simulink model "protocol"  (R2021b)
settings: Solver=FixedStepAuto  StartTime=0.0  StopTime=10.0  RelTol=1e-3
settings Model: Creator=marco  LastModifiedBy=makev
settings ModelReferenceCC: UpdateModelReferenceTargets=IfOutOfDate
settings ConfigComp: DVTestSuiteOptimization=Auto  DVDetectOutOfBounds=on  DVModelReferenceHarness=on

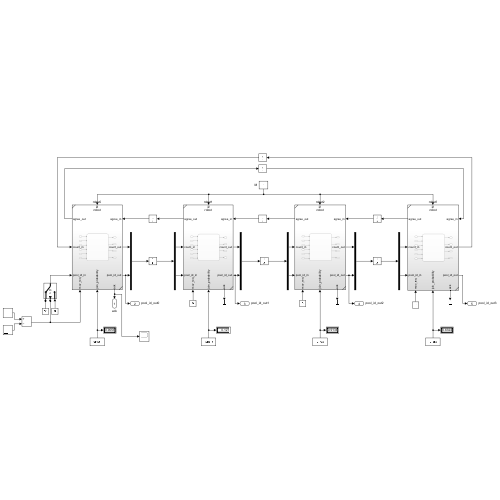
[thumbnail: Simulink's stored preview of the top-level diagram]
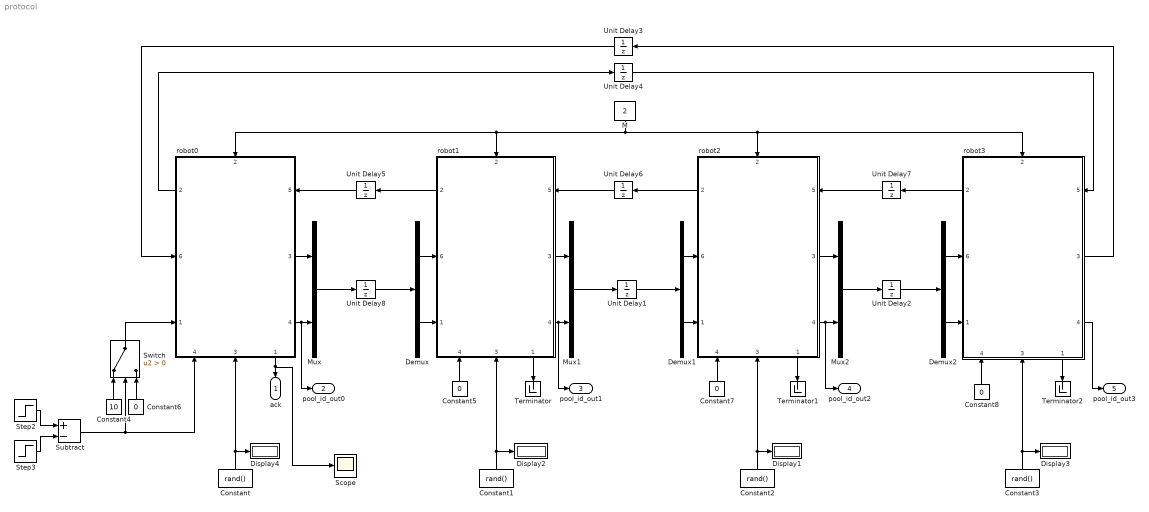
== system protocol ==
  Constant{,1..3} (4 alike) : Constant  Value=rand()
  Constant4 : Constant  Value=10
  Constant{5..8} (4 alike) : Constant  Value=0
  Demux : Demux  Outputs=2
  Demux1 : Demux  Outputs=2
  Demux2 : Demux  Outputs=2
  Display{1..4} (4 alike) : Display
  M : Constant  Value=2
  Mux : Mux  Inputs=2
  Mux1 : Mux  Inputs=2
  Mux2 : Mux  Inputs=2
  Scope : Scope
  Step2 : Step  SampleTime=.2
  Step3 : Step  Time=1.2  SampleTime=.2
  Subtract : Sum  Inputs=+-
  Switch : Switch  Criteria=u2 > Threshold
  Terminator : Terminator
  Terminator1 : Terminator
  Terminator2 : Terminator
  Unit Delay{1..8} (8 alike) : UnitDelay  SampleTime=-1  HasFrameUpgradeWarning=on
  robot{0..3} (4 alike) : Subsystem  ReferencedSubsystem=robot
      robot0 settings: PortSchema="{\"entries\":[{\"content\":{\"sides\":[{\"content\":{\"connectorIds\":[\"Out2\",\"In6\",\"In1\"]},\"type\":\"ConnectorPlacement.EquallySpacedRectSide\",\"uuid\":\"c2973ddf-8c1f-4294-82f9-250d4d64bc41\"},{\"content\":{\"connectorIds\":[\"In5\",\"Out3\",\"Out4\"],\"side\":\"RIGHT\"},\"type\":\"ConnectorPlacement.EquallySpacedRectSide\",\"uuid\":\"34f58778-6b96-4f4c-9fc2-6c1c729063a8\"},{\"content\":{\"connectorIds\":[\"In2\"],\"side\":\"TOP\"},\"type\":\"ConnectorPlacement.EquallySpacedRectSide\",\"uuid\":\"80e910fc-ff47-444b-b672-e337659921ae\"},{\"content\":{\"connectorIds\":[\"In4\",\"In3\",\"Out1\"],\"side\":\"BOTTOM\"},\"type\":\"ConnectorPlacement.EquallySpacedRectSide\",\"uuid\":\"4c5b4a6c-4ee5-43a5-b389-1d5635d4cbda\"}]},\"type\":\"ConnectorPlacement.EquallySpacedConnector\",\"uuid\":\"573bf93a-1f25-4267-812c-06cdd99b033a\"}],\"packageUris\":[\"http://schema.mathworks.com/mf0/Connector/R2020b\"],\"version\":\"1.0\"}"
      robot1 settings: PortSchema="{\"entries\":[{\"content\":{\"sides\":[{\"content\":{\"connectorIds\":[\"Out2\",\"In6\",\"In1\"]},\"type\":\"ConnectorPlacement.EquallySpacedRectSide\",\"uuid\":\"c2973ddf-8c1f-4294-82f9-250d4d64bc41\"},{\"content\":{\"connectorIds\":[\"In5\",\"Out3\",\"Out4\"],\"side\":\"RIGHT\"},\"type\":\"ConnectorPlacement.EquallySpacedRectSide\",\"uuid\":\"34f58778-6b96-4f4c-9fc2-6c1c729063a8\"},{\"content\":{\"connectorIds\":[\"In2\"],\"side\":\"TOP\"},\"type\":\"ConnectorPlacement.EquallySpacedRectSide\",\"uuid\":\"80e910fc-ff47-444b-b672-e337659921ae\"},{\"content\":{\"connectorIds\":[\"In4\",\"In3\",\"Out1\"],\"side\":\"BOTTOM\"},\"type\":\"ConnectorPlacement.EquallySpacedRectSide\",\"uuid\":\"e4e016b7-b76e-4e62-a0db-89e9df8dea8e\"}]},\"type\":\"ConnectorPlacement.EquallySpacedConnector\",\"uuid\":\"573bf93a-1f25-4267-812c-06cdd99b033a\"}],\"packageUris\":[\"http://schema.mathworks.com/mf0/Connector/R2020b\"],\"version\":\"1.0\"}"
      robot2 settings: PortSchema="{\"entries\":[{\"content\":{\"sides\":[{\"content\":{\"connectorIds\":[\"Out2\",\"In6\",\"In1\"]},\"type\":\"ConnectorPlacement.EquallySpacedRectSide\",\"uuid\":\"c2973ddf-8c1f-4294-82f9-250d4d64bc41\"},{\"content\":{\"connectorIds\":[\"In5\",\"Out3\",\"Out4\"],\"side\":\"RIGHT\"},\"type\":\"ConnectorPlacement.EquallySpacedRectSide\",\"uuid\":\"34f58778-6b96-4f4c-9fc2-6c1c729063a8\"},{\"content\":{\"connectorIds\":[\"In2\"],\"side\":\"TOP\"},\"type\":\"ConnectorPlacement.EquallySpacedRectSide\",\"uuid\":\"80e910fc-ff47-444b-b672-e337659921ae\"},{\"content\":{\"connectorIds\":[\"In4\",\"In3\",\"Out1\"],\"side\":\"BOTTOM\"},\"type\":\"ConnectorPlacement.EquallySpacedRectSide\",\"uuid\":\"2cd792df-4aad-4f2e-80f9-e48174994b0d\"}]},\"type\":\"ConnectorPlacement.EquallySpacedConnector\",\"uuid\":\"573bf93a-1f25-4267-812c-06cdd99b033a\"}],\"packageUris\":[\"http://schema.mathworks.com/mf0/Connector/R2020b\"],\"version\":\"1.0\"}"
      robot3 settings: PortSchema="{\"entries\":[{\"content\":{\"sides\":[{\"content\":{\"connectorIds\":[\"Out2\",\"In6\",\"In1\"]},\"type\":\"ConnectorPlacement.EquallySpacedRectSide\",\"uuid\":\"c2973ddf-8c1f-4294-82f9-250d4d64bc41\"},{\"content\":{\"connectorIds\":[\"In5\",\"Out3\",\"Out4\"],\"side\":\"RIGHT\"},\"type\":\"ConnectorPlacement.EquallySpacedRectSide\",\"uuid\":\"34f58778-6b96-4f4c-9fc2-6c1c729063a8\"},{\"content\":{\"connectorIds\":[\"In2\"],\"side\":\"TOP\"},\"type\":\"ConnectorPlacement.EquallySpacedRectSide\",\"uuid\":\"80e910fc-ff47-444b-b672-e337659921ae\"},{\"content\":{\"connectorIds\":[\"In4\",\"In3\",\"Out1\"],\"side\":\"BOTTOM\"},\"type\":\"ConnectorPlacement.EquallySpacedRectSide\",\"uuid\":\"e1d2a9a1-3695-4a7a-a698-108fcecfffe2\"}]},\"type\":\"ConnectorPlacement.EquallySpacedConnector\",\"uuid\":\"573bf93a-1f25-4267-812c-06cdd99b033a\"}],\"packageUris\":[\"http://schema.mathworks.com/mf0/Connector/R2020b\"],\"version\":\"1.0\"}"
  ack : Outport
  pool_id_out0 : Outport  Port=2
  pool_id_out1 : Outport  Port=3
  pool_id_out2 : Outport  Port=4
  pool_id_out3 : Outport  Port=5
  wires:
  robot0/1 -> Scope/1, ack/1
  robot1/1 -> Terminator/1
  robot2/1 -> Terminator1/1
  robot3/1 -> Terminator2/1
  robot3/3 -> Unit Delay3/1
  robot1/2 -> Unit Delay5/1
  robot2/2 -> Unit Delay6/1
  robot3/2 -> Unit Delay7/1
  robot0/2 -> Unit Delay4/1
  Constant1/1 -> robot1/3, Display2/1
  Constant2/1 -> robot2/3, Display1/1
  Unit Delay3/1 -> robot0/6
  Unit Delay4/1 -> robot3/5
  Unit Delay5/1 -> robot0/5
  Unit Delay6/1 -> robot1/5
  Unit Delay7/1 -> robot2/5
  Constant/1 -> robot0/3, Display4/1
  Subtract/1 -> Switch/2, robot0/4
  Constant3/1 -> Display3/1, robot3/3
  Constant7/1 -> robot2/4
  Constant8/1 -> robot3/4
  Constant5/1 -> robot1/4
  M/1 -> robot2/2, robot3/2, robot0/2, robot1/2
  Switch/1 -> robot0/1
  robot3/4 -> pool_id_out3/1
  robot0/3 -> Mux/1
  robot0/4 -> pool_id_out0/1, Mux/2
  Demux/1 -> robot1/6
  Demux/2 -> robot1/1
  Mux/1 -> Unit Delay8/1
  Unit Delay8/1 -> Demux/1
  Demux1/1 -> robot2/6
  Mux1/1 -> Unit Delay1/1
  Unit Delay1/1 -> Demux1/1
  Demux1/2 -> robot2/1
  robot1/3 -> Mux1/1
  robot1/4 -> pool_id_out1/1, Mux1/2
  Mux2/1 -> Unit Delay2/1
  Unit Delay2/1 -> Demux2/1
  robot2/3 -> Mux2/1
  robot2/4 -> pool_id_out2/1, Mux2/2
  Demux2/1 -> robot3/6
  Demux2/2 -> robot3/1
  Constant4/1 -> Switch/1
  Constant6/1 -> Switch/3
  Step2/1 -> Subtract/1
  Step3/1 -> Subtract/2
